simulink model "lab6"  (R2018a)
settings: Solver=ode45  StartTime=0.0  StopTime=15  MaxStep=2^-5  RelTol=1e-3
settings Model: Creator=gigol  LastModifiedBy=gigol

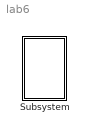
== system lab6 ==
  Subsystem : Subsystem  mask{g=9.81, k1=2, k2=1, m1=1, m2=2, l1=1, l2=2, fi10=80, fi20=150}

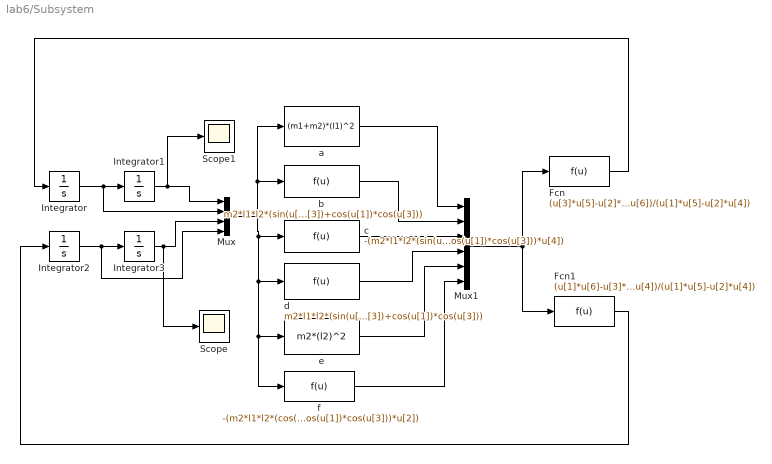
== system lab6/Subsystem ==
  Fcn : Fcn  Expr=(u[3]*u[5]-u[2]*u[6])/(u[1]*u[5]-u[2]*u[4])
  Fcn1 : Fcn  Expr=(u[1]*u[6]-u[3]*u[4])/(u[1]*u[5]-u[2]*u[4])
  Integrator : Integrator
  Integrator1 : Integrator  InitialCondition=(fi10*pi)/180
  Integrator2 : Integrator
  Integrator3 : Integrator  InitialCondition=(fi20*pi)/180
  Mux : Mux
  Mux1 : Mux  Inputs=6
  Scope : Scope
  Scope1 : Scope
  a : Fcn  Expr=(m1+m2)*(l1)^2
  b : Fcn  Expr=m2*l1*l2*(sin(u[1])*sin(u[3])+cos(u[1])*cos(u[3]))
  c : Fcn  Expr=-(m2*l1*l2*(sin(u[1])*cos(u[3])-cos(u[1])*sin(u[3]))*(u[4])^2 + (m1+m2)*g*(l1)*sin(u[1])+k1*(l1)^2*u[2]+k2*l1*l2*(sin(u[1])*sin(u[3])+cos(u[1])*cos(u[3]))*u[4])
  d : Fcn  Expr=m2*l1*l2*(sin(u[1])*sin(u[3])+cos(u[1])*cos(u[3]))
  e : Fcn  Expr=m2*(l2)^2
  f : Fcn  Expr=-(m2*l1*l2*(cos(u[1])*sin(u[3])-sin(u[1])*cos(u[3]))*(u[2])^2 + m2*g*l2*sin(u[3])+k2*(l2)^2*u[4]+k2*l1*l2*(sin(u[1])*sin(u[3])+cos(u[1])*cos(u[3]))*u[2])
  wires:
  Mux1/1 -> Fcn/1, Fcn1/1
  d/1 -> Mux1/4
  Integrator3/1 -> Scope/1, Mux/3
  Integrator1/1 -> Scope1/1, Mux/1
  e/1 -> Mux1/5
  Mux/1 -> f/1, e/1, d/1, c/1, b/1, a/1
  Integrator/1 -> Mux/2, Integrator1/1
  Integrator2/1 -> Mux/4, Integrator3/1
  Fcn1/1 -> Integrator2/1
  a/1 -> Mux1/1
  b/1 -> Mux1/2
  c/1 -> Mux1/3
  Fcn/1 -> Integrator/1
  f/1 -> Mux1/6
